simulink model "lab3"  (R2018b)
settings: Solver=ode45  StartTime=0.0  StopTime=200  FixedStep=0.1  MaxStep=0.1  RelTol=1e-3
undefined symbols (not defined in the file or in its folder): alpha, Kr, Td, Ti
settings Model: Creator=FetCatz  LastModifiedBy=FetCatz
settings SolverCC: AutoInsertRateTranBlk=on

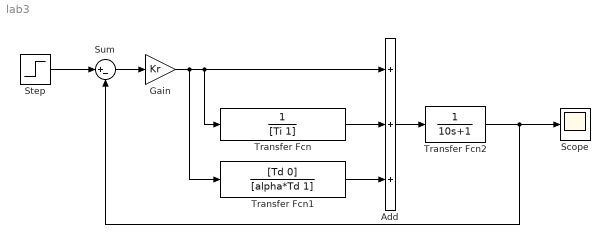
== system lab3 ==
  Add : Sum  Inputs=+++
  Gain : Gain  Gain=Kr
  Scope : Scope
  Step : Step  Time=0  SampleTime=0
  Sum : Sum  Inputs=|+-
  Transfer Fcn : TransferFcn  Denominator=[Ti 1]
  Transfer Fcn1 : TransferFcn  Numerator=[Td 0]  Denominator=[alpha*Td 1]
  Transfer Fcn2 : TransferFcn  Denominator=[10 1]
  wires:
  Step/1 -> Sum/1
  Sum/1 -> Gain/1
  Gain/1 -> Add/1, Transfer Fcn/1, Transfer Fcn1/1
  Transfer Fcn/1 -> Add/2
  Transfer Fcn1/1 -> Add/3
  Add/1 -> Transfer Fcn2/1
  Transfer Fcn2/1 -> Sum/2, Scope/1
